simulink model "rasoc_tesis_v4"  (R2021a)
settings: Solver=FixedStepAuto  StartTime=0.0  StopTime=inf  FixedStep=0.01  RelTol=1e-3
values from neighbouring files (symbols this model uses):
  a = 0.445    [param_tesis.m]
  a_max = v_max/dt    (= 0.8)    [param_tesis.m]
  alt_z = 0    [param_tesis.m]
  B = 0.5    [param_tesis.m]
  currentPose = [47 43.5 0]    [param_tesis.m]
  efic_red = 0.95    [param_tesis.m]
  goalPose = [1.5 5 pi/2]    [param_tesis.m]
  gpsBasePose = [1 44]    [param_tesis.m]
  kb = 8.93*(3/(1000*pi))    (= 0.00852752185086)    [param_tesis.m]
  kt = 0.077*sqrt(2)*3    [param_tesis.m]
  L = 0.55    [param_tesis.m]
  m_uva = 0    [param_tesis.m]
  n = 16    [param_tesis.m]
  r = 0.125    [param_tesis.m]
  Ra = Vnom/Ipeak    (= 14.2857142857)    [param_tesis.m]
  Rp = Ra*20    (= 285.714285714)    [param_tesis.m]
  t_lpf = 1/200    (= 0.005)    [param_tesis.m]
  tau_max = 5    [param_tesis.m]
  v_max = 0.8    [param_tesis.m]
  Vnom = 310    [param_tesis.m]
  w_max = 0.5    [param_tesis.m]
  waypoints = [currentPose(1), currentPose(2) ... (first row only)    [AstarHybrid_fn.m]    (also in param_tesis.m = AstarHybrid_fn(currentPose, goalPose))
undefined symbols (not defined in the file or in its folder): angular, DiscIntNeverNeededParam, Earth, linear, startTheta, startX, startY, WGS84
libraries: ros2lib x10, simulink x5, mobileRoboticsTrainingLib x3, robotmobilelib x2, pid_lib x2, robotalgslib x2, aerolibtransform2 x2, dspstat3 x1
(part 2 of 2)

== system rasoc_tesis_v4/Subsystem1/Tensión y Motores/Modulador de Tensión ==
  Va_mL* : Inport
  Va_mR* : Inport  Port=2
  Filtro : StateSpace  A=[-1/t_lpf]  B=[1]  C=[1/t_lpf]  D=[0]  InitialCondition=0
  Filtro PB 1° Orden : StateSpace  A=[-1/t_lpf]  B=[1]  C=[1/t_lpf]  D=[0]  InitialCondition=0
  Saturación : Saturate  UpperLimit=Vnom  LowerLimit=-Vnom
  Saturation : Saturate  UpperLimit=Vnom  LowerLimit=-Vnom
  Va_mL : Outport
  Va_mR : Outport  Port=2
  wires:
  Filtro PB 1° Orden/1 -> Saturación/1
  Filtro/1 -> Saturation/1
  Saturation/1 -> Va_mR/1
  Saturación/1 -> Va_mL/1
  Va_mL*/1 -> Filtro PB 1° Orden/1
  Va_mR*/1 -> Filtro/1

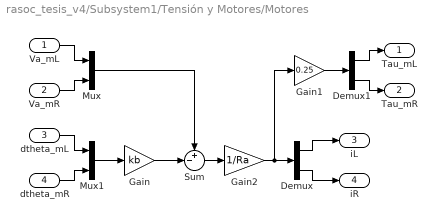
== system rasoc_tesis_v4/Subsystem1/Tensión y Motores/Motores ==
  Va_mL : Inport
  Va_mR : Inport  Port=2
  dtheta_mL : Inport  Port=3
  dtheta_mR : Inport  Port=4
  Demux : Demux  Outputs=2
  Demux1 : Demux  Outputs=2
  Gain : Gain  Gain=kb
  Gain1 : Gain  Gain=0.25
  Gain2 : Gain  Gain=1/Ra
  Mux : Mux  Inputs=2
  Mux1 : Mux  Inputs=2
  Sum : Sum  Inputs=+-|
  Tau_mL : Outport
  Tau_mR : Outport  Port=2
  iL : Outport  Port=3
  iR : Outport  Port=4
  wires:
  Demux/2 -> iR/1
  Va_mL/1 -> Mux/1
  Demux/1 -> iL/1
  dtheta_mR/1 -> Mux1/2
  dtheta_mL/1 -> Mux1/1
  Demux1/2 -> Tau_mR/1
  Demux1/1 -> Tau_mL/1
  Va_mR/1 -> Mux/2
  Mux1/1 -> Gain/1
  Gain1/1 -> Demux1/1
  Gain/1 -> Sum/2
  Mux/1 -> Sum/1
  Sum/1 -> Gain2/1
  Gain2/1 -> Gain1/1, Demux/1

== system rasoc_tesis_v4/Subsystem1/Torque y Corriente/Desacople ==
  Va_mL*' : Inport
  Va_mR*' : Inport  Port=2
  dtheta_mL^ : Inport  Port=3
  dtheta_mR^ : Inport  Port=4
  Demux : Demux  Outputs=2
  Gain1 : Gain  Gain=kb
  Mux : Mux  Inputs=2
  Mux1 : Mux  Inputs=2
  Sum : Sum  Inputs=|++
  Va_mL* : Outport
  Va_mR* : Outport  Port=2
  wires:
  dtheta_mL^/1 -> Mux1/1
  Mux1/1 -> Gain1/1
  Va_mR*'/1 -> Mux/2
  Demux/1 -> Va_mL*/1
  Gain1/1 -> Sum/2
  Mux/1 -> Sum/1
  Sum/1 -> Demux/1
  Va_mL*'/1 -> Mux/1
  Demux/2 -> Va_mR*/1
  dtheta_mR^/1 -> Mux1/2

== system rasoc_tesis_v4/Subsystem1/Torque y Corriente/Modulador de Corriente ==
  "iL* " : Inport
  iR* : Inport  Port=2
  iL^ : Inport  Port=3
  iR^ : Inport  Port=4
  Control Proporcional : Gain  Gain=Rp
  Demux : Demux  Outputs=2
  Mux : Mux  Inputs=2
  Sum : Sum  Inputs=-+|
  Sum1 : Sum  Inputs=|+-
  Va_mL*' : Outport
  Va_mR*' : Outport  Port=2
  wires:
  iL^/1 -> Sum/1
  "iL* "/1 -> Sum/2
  iR*/1 -> Sum1/1
  iR^/1 -> Sum1/2
  Mux/1 -> Control Proporcional/1
  Control Proporcional/1 -> Demux/1
  Sum/1 -> Mux/1
  Sum1/1 -> Mux/2
  Demux/1 -> Va_mL*'/1
  Demux/2 -> Va_mR*'/1

== system rasoc_tesis_v4/Subsystem1/Torque y Corriente/Modulador de Torque ==
  Tau_mL* : Inport
  Tau_mR* : Inport  Port=2
  Demux : Demux  Outputs=2
  Gain : Gain  Gain=1/kt
  Mux : Mux  Inputs=2
  Saturation : Saturate  UpperLimit=tau_max  LowerLimit=-tau_max
  iL* : Outport
  iR* : Outport  Port=2
  wires:
  Tau_mL*/1 -> Mux/1
  Demux/2 -> iR*/1
  Demux/1 -> iL*/1
  Gain/1 -> Demux/1
  Tau_mR*/1 -> Mux/2
  Mux/1 -> Saturation/1
  Saturation/1 -> Gain/1

== system rasoc_tesis_v4/Subsystem4/Local Navigation/Path Following ==
  SteeringDirection : Inport
  AngularVelocity : Inport  Port=2
  Action Port : ActionPort  ActionPortLabel=else
  Compute Angular Velocity : MATLAB Function  TreatAsAtomicUnit=on
  Constant : Constant  Value=0
  MaxAngularVelocity : Constant  Value=w_max
  Subtract : Sum  Inputs=+-
  dV : Outport  VectorParamsAs1DForOutWhenUnconnected=off
  dW : Outport  Port=2  VectorParamsAs1DForOutWhenUnconnected=off
  wires:
  Constant/1 -> dV/1
  MaxAngularVelocity/1 -> Compute Angular Velocity/2(wMax)
  SteeringDirection/1 -> Compute Angular Velocity/1(steeringDir)
  Subtract/1 -> dW/1
  Compute Angular Velocity/1(w) -> Subtract/1
  AngularVelocity/1 -> Subtract/2

== system rasoc_tesis_v4/Subsystem4/Local Navigation/Recovery ==
  LinVel : Inport
  AngVel : Inport  Port=2
  Action Port : ActionPort  ActionPortLabel=if(u1 == 1)
  Constant1 : Constant  Value=0.2
  Gain : Gain  Gain=-1
  Subtract : Sum  Inputs=+-
  dV : Outport  VectorParamsAs1DForOutWhenUnconnected=off
  dW : Outport  Port=2  VectorParamsAs1DForOutWhenUnconnected=off
  wires:
  LinVel/1 -> Gain/1
  Gain/1 -> dV/1
  Constant1/1 -> Subtract/1
  AngVel/1 -> Subtract/2
  Subtract/1 -> dW/1

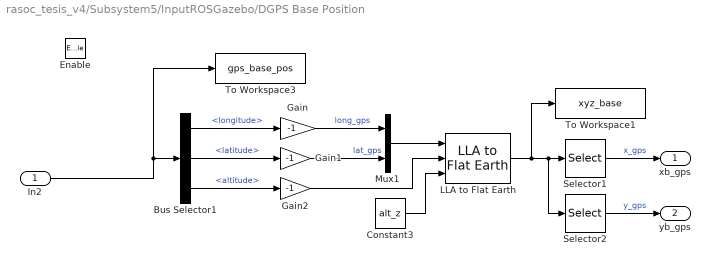
== system rasoc_tesis_v4/Subsystem5/InputROSGazebo/DGPS Base Position ==
  In2 : Inport
  Enable : EnablePort
  Bus Selector1 : BusSelector  OutputSignals=longitude,latitude,altitude
  Constant3 : Constant  Value=alt_z
  Gain : Gain  Gain=-1
  Gain1 : Gain  Gain=-1
  Gain2 : Gain  Gain=-1
  LLA to Flat Earth : aerolibtransform2/LLA to Flat Earth  units=Metric (MKS)  ptype=Earth (WGS84)  F=1/298.257223563  R=6378137  refPosPort=off  LL0=[0 0]  psi=0
      settings: SourceProductBaseCode=AE
  Mux1 : Mux  Inputs=2
  Selector1 : Selector  InputPortWidth=3  IndexOptions=Index vector (dialog)  Indices=[1]  OutputSizes=1
  Selector2 : Selector  InputPortWidth=3  IndexOptions=Index vector (dialog)  Indices=[2]  OutputSizes=1
  To Workspace1 : ToWorkspace  VariableName=xyz_base  SampleTime=-1
  To Workspace3 : ToWorkspace  VariableName=gps_base_pos  SaveFormat=Timeseries  SampleTime=-1
  xb_gps : Outport
  yb_gps : Outport  Port=2
  wires:
  In2/1 -> Bus Selector1/1, To Workspace3/1
  Bus Selector1/2 -> Gain1/1  "<latitude>"
  Bus Selector1/1 -> Gain/1  "<longitude>"
  Gain2/1 -> LLA to Flat Earth/2
  Mux1/1 -> LLA to Flat Earth/1
  LLA to Flat Earth/1 -> Selector2/1, Selector1/1, To Workspace1/1
  Gain/1 -> Mux1/1  "long_gps"
  Gain1/1 -> Mux1/2  "lat_gps"
  Constant3/1 -> LLA to Flat Earth/3
  Bus Selector1/3 -> Gain2/1  "<altitude>"
  Selector1/1 -> xb_gps/1  "x_gps"
  Selector2/1 -> yb_gps/1  "y_gps"

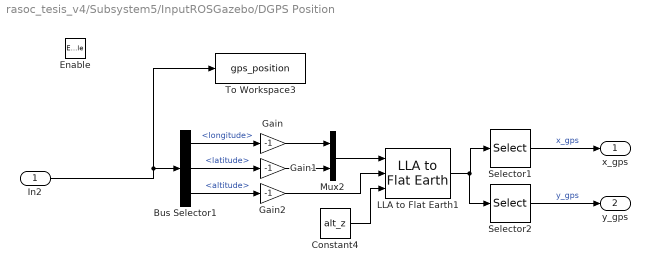
== system rasoc_tesis_v4/Subsystem5/InputROSGazebo/DGPS Position ==
  In2 : Inport
  Enable : EnablePort
  Bus Selector1 : BusSelector  OutputSignals=longitude,latitude,altitude
  Constant4 : Constant  Value=alt_z
  Gain : Gain  Gain=-1
  Gain1 : Gain  Gain=-1
  Gain2 : Gain  Gain=-1
  LLA to Flat Earth1 : aerolibtransform2/LLA to Flat Earth  units=Metric (MKS)  ptype=Earth (WGS84)  F=1/298.257223563  R=6378137  refPosPort=off  LL0=[0 0]  psi=0
      settings: SourceProductBaseCode=AE
  Mux2 : Mux  Inputs=2
  Selector1 : Selector  InputPortWidth=3  IndexOptions=Index vector (dialog)  Indices=[1]  OutputSizes=1
  Selector2 : Selector  InputPortWidth=3  IndexOptions=Index vector (dialog)  Indices=[2]  OutputSizes=1
  To Workspace3 : ToWorkspace  VariableName=gps_position  SaveFormat=Timeseries  SampleTime=-1
  x_gps : Outport
  y_gps : Outport  Port=2
  wires:
  Bus Selector1/1 -> Gain/1  "<longitude>"
  Bus Selector1/2 -> Gain1/1  "<latitude>"
  In2/1 -> To Workspace3/1, Bus Selector1/1
  Bus Selector1/3 -> Gain2/1  "<altitude>"
  Constant4/1 -> LLA to Flat Earth1/3
  Mux2/1 -> LLA to Flat Earth1/1
  Gain2/1 -> LLA to Flat Earth1/2
  Gain1/1 -> Mux2/2
  Gain/1 -> Mux2/1
  LLA to Flat Earth1/1 -> Selector2/1, Selector1/1
  Selector1/1 -> x_gps/1  "x_gps"
  Selector2/1 -> y_gps/1  "y_gps"

== system rasoc_tesis_v4/Subsystem5/InputROSGazebo/DGPS Vel ==
  In1 : Inport
  Enable : EnablePort
  Bus Selector3 : BusSelector  OutputSignals=vector.x,vector.y
  Gain : Gain  Gain=-1
  Gain1 : Gain  Gain=-1
  To Workspace6 : ToWorkspace  VariableName=gps_velocity  SaveFormat=Timeseries  SampleTime=-1
  dx_gps : Outport
  dy_gps : Outport  Port=2
  wires:
  Bus Selector3/1 -> Gain/1  "<x>"
  In1/1 -> To Workspace6/1, Bus Selector3/1
  Bus Selector3/2 -> Gain1/1  "<y>"
  Gain/1 -> dx_gps/1
  Gain1/1 -> dy_gps/1

== system rasoc_tesis_v4/Subsystem5/InputROSGazebo/GPS2ROS ==
  x_gps : Inport
  y_gps : Inport  Port=2
  v_gps : Inport  Port=3
  w_gps : Inport  Port=4
  Action Port : ActionPort  ActionPortLabel=if(u1 == 1)
  x_ros : Outport  VectorParamsAs1DForOutWhenUnconnected=off
  y_ros : Outport  Port=2  VectorParamsAs1DForOutWhenUnconnected=off
  v_ros : Outport  Port=3  VectorParamsAs1DForOutWhenUnconnected=off
  w_ros : Outport  Port=4  VectorParamsAs1DForOutWhenUnconnected=off
  wires:
  x_gps/1 -> x_ros/1
  y_gps/1 -> y_ros/1
  w_gps/1 -> w_ros/1
  v_gps/1 -> v_ros/1

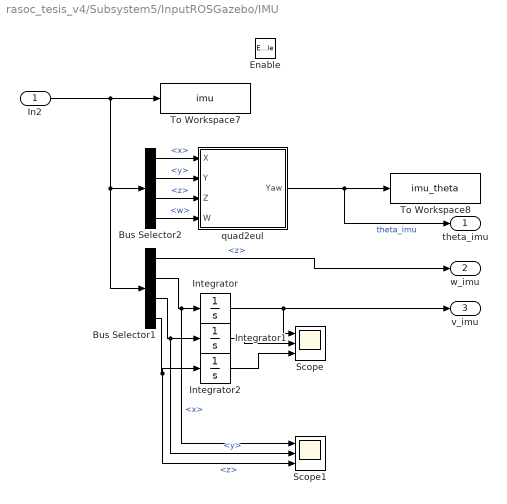
== system rasoc_tesis_v4/Subsystem5/InputROSGazebo/IMU ==
  In2 : Inport
  Enable : EnablePort
  Bus Selector1 : BusSelector  OutputSignals=angular_velocity.z,linear_acceleration.x,linear_acceleration.y,linear_acceleration.z
  Bus Selector2 : BusSelector  OutputSignals=orientation.x,orientation.y,orientation.z,orientation.w
  Integrator : Integrator
  Integrator1 : Integrator
  Integrator2 : Integrator
  Scope : Scope  NumInputPorts=3
  Scope1 : Scope  NumInputPorts=3
  To Workspace7 : ToWorkspace  VariableName=imu  SaveFormat=Timeseries  SampleTime=-1
  To Workspace8 : ToWorkspace  VariableName=imu_theta  SaveFormat=Timeseries  SampleTime=-1
  quad2eul : MATLAB Function  TreatAsAtomicUnit=on
  theta_imu : Outport
  w_imu : Outport  Port=2
  v_imu : Outport  Port=3
  wires:
  Bus Selector2/3 -> quad2eul/3(Z)  "<z>"
  quad2eul/1(Yaw) -> theta_imu/1, To Workspace8/1  "theta_imu"
  In2/1 -> Bus Selector1/1, Bus Selector2/1, To Workspace7/1
  Bus Selector2/1 -> quad2eul/1(X)  "<x>"
  Bus Selector2/4 -> quad2eul/4(W)  "<w>"
  Bus Selector2/2 -> quad2eul/2(Y)  "<y>"
  Bus Selector1/1 -> w_imu/1  "<z>"
  Bus Selector1/2 -> Scope1/1, Integrator/1  "<x>"
  Integrator/1 -> Scope/1, v_imu/1
  Bus Selector1/3 -> Scope1/2, Integrator1/1  "<y>"
  Bus Selector1/4 -> Scope1/3, Integrator2/1  "<z>"
  Integrator1/1 -> Scope/2
  Integrator2/1 -> Scope/3

== system rasoc_tesis_v4/Subsystem5/InputROSGazebo/IMU2ROS ==
  theta_imu : Inport
  Action Port : ActionPort  ActionPortLabel=if(u1 == 1)
  theta_ros : Outport  VectorParamsAs1DForOutWhenUnconnected=off
  wires:
  theta_imu/1 -> theta_ros/1

== system rasoc_tesis_v4/Subsystem5/InputROSGazebo/LIDAR ==
  In1 : Inport
  MATLAB Function : MATLAB Function  TreatAsAtomicUnit=on
  To Workspace1 : ToWorkspace  VariableName=Lidar  SaveFormat=Timeseries  SampleTime=-1
  Ranges : Outport
  Angles : Outport  Port=2
  wires:
  In1/1 -> To Workspace1/1, MATLAB Function/1(LaserScanMsg)
  MATLAB Function/2(Angles) -> Angles/1
  MATLAB Function/1(Ranges) -> Ranges/1

== system rasoc_tesis_v4/Subsystem5/InputROSGazebo/ODOM2ROS ==
  x_odom : Inport
  y_odom : Inport  Port=2
  v_odom : Inport  Port=3
  w_odom : Inport  Port=4
  Action Port : ActionPort  ActionPortLabel=else
  x_ros : Outport  VectorParamsAs1DForOutWhenUnconnected=off
  y_ros : Outport  Port=2  VectorParamsAs1DForOutWhenUnconnected=off
  v_ros : Outport  Port=3  VectorParamsAs1DForOutWhenUnconnected=off
  w_ros : Outport  Port=4  VectorParamsAs1DForOutWhenUnconnected=off
  wires:
  x_odom/1 -> x_ros/1
  y_odom/1 -> y_ros/1
  v_odom/1 -> v_ros/1
  w_odom/1 -> w_ros/1

== system rasoc_tesis_v4/Subsystem5/InputROSGazebo/ODOM2ROS_theta ==
  theta_odom : Inport
  Action Port : ActionPort  ActionPortLabel=else
  theta_ros : Outport  VectorParamsAs1DForOutWhenUnconnected=off
  wires:
  theta_odom/1 -> theta_ros/1

== system rasoc_tesis_v4/Subsystem5/InputROSGazebo/Odometry ==
  In1 : Inport
  Bus Selector : BusSelector  OutputSignals=pose.pose.position.x,pose.pose.position.y,pose.pose.orientation.x,pose.pose.orientation.y,pose.pose.orientation.z,pose.pose.orientation.w
  Bus Selector1 : BusSelector  OutputSignals=twist.twist.linear.x,twist.twist.angular.z
  XY ODOM : simulink/Sinks/XY Graph  Commented=on  xmin=0  xmax=50  ymin=-5  ymax=50  st=-1
  quad2eul : MATLAB Function  TreatAsAtomicUnit=on
  x_odom : Outport
  y_odom : Outport  Port=2
  theta_odom : Outport  Port=3
  v_odom : Outport  Port=4
  w_odom : Outport  Port=5
  wires:
  Bus Selector/5 -> quad2eul/3(Z)  "<z>"
  Bus Selector/1 -> x_odom/1, XY ODOM/1  "<x>"
  quad2eul/1(Yaw) -> theta_odom/1
  Bus Selector/3 -> quad2eul/1(X)  "<x>"
  Bus Selector1/1 -> v_odom/1  "<x>"
  Bus Selector/2 -> y_odom/1, XY ODOM/2  "<y>"
  In1/1 -> Bus Selector/1, Bus Selector1/1
  Bus Selector1/2 -> w_odom/1  "<z>"
  Bus Selector/6 -> quad2eul/4(W)  "<w>"
  Bus Selector/4 -> quad2eul/2(Y)  "<y>"

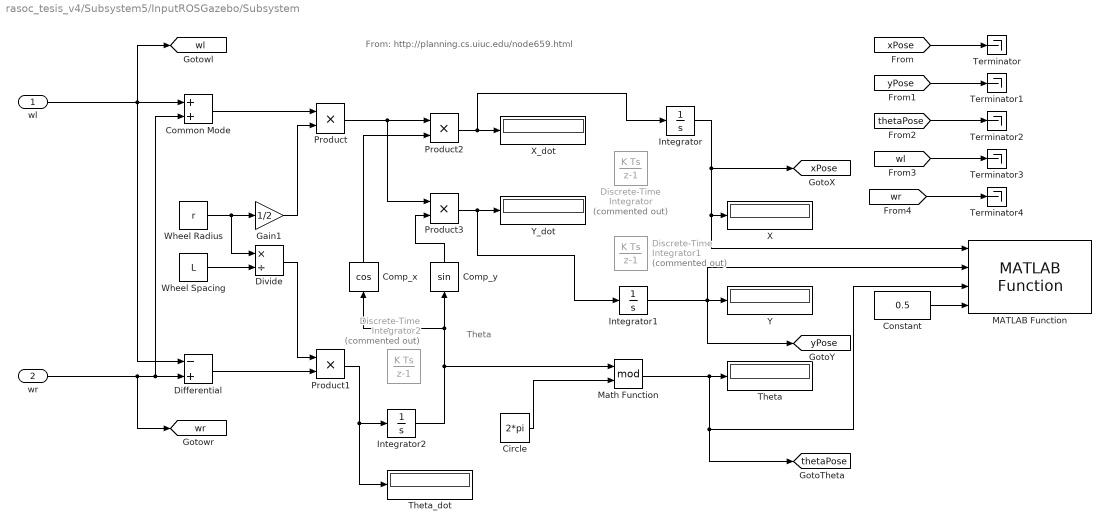
== system rasoc_tesis_v4/Subsystem5/InputROSGazebo/Subsystem ==
  note: Theta
  note: From: http://planning.cs.uiuc.edu/node659.html
  wl : Inport
  wr : Inport  Port=2
  Circle : Constant  Value=2*pi
  Common Mode : Sum
  Comp_x : Trigonometry  Operator=cos
  Comp_y : Trigonometry
  Constant : Constant  Value=0.5
  Differential : Sum  Inputs=-+
  Discrete-Time Integrator : DiscreteIntegrator  Commented=on  InitialCondition=startX  SampleTime=-1  ICPrevOutput=DiscIntNeverNeededParam  ICPrevScaledInput=DiscIntNeverNeededParam
  Discrete-Time Integrator1 : DiscreteIntegrator  Commented=on  InitialCondition=startY  SampleTime=-1  ICPrevOutput=DiscIntNeverNeededParam  ICPrevScaledInput=DiscIntNeverNeededParam
  Discrete-Time Integrator2 : DiscreteIntegrator  Commented=on  InitialCondition=startTheta*(pi/180)  SampleTime=-1  ICPrevOutput=DiscIntNeverNeededParam  ICPrevScaledInput=DiscIntNeverNeededParam
  Divide : Product  Inputs=*/
  Gain1 : Gain  Gain=1/2
  Integrator : Integrator  InitialCondition=currentPose(1)
  Integrator1 : Integrator  InitialCondition=currentPose(2)
  Integrator2 : Integrator  InitialCondition=currentPose(3)
  MATLAB Function : mobileRoboticsTrainingLib/Robot Simulator/MATLAB Function  SystemSampleTime=-1  VariantActivationTime=update diagram  Latency=0  AutoFrameSizeCalculation=off
      settings: SourceProductName=Mobile Robotics Training Library
  Math Function : Math  Operator=mod  SignedPower=on  SaturateOnIntegerOverflow=on
  Product{,1..3} (4 alike) : Product  RndMeth=Zero
  Terminator{,1..4} (5 alike) : Terminator
  Theta : Display
  Theta_dot : Display
  Wheel Radius : Constant  Value=r
  Wheel Spacing : Constant  Value=L
  X : Display
  X_dot : Display
  Y : Display
  Y_dot : Display
  tag scope: thetaPose=global, wl=global, wr=global, xPose=global, yPose=global
  wires:
  Common Mode/1 -> Product/1
  Math Function/1 -> [thetaPose], MATLAB Function/3, Theta/1
  wl/1 -> [wl], Common Mode/1, Differential/1
  Integrator2/1 -> Math Function/1, Comp_x/1, Comp_y/1
  Divide/1 -> Product1/1
  Product3/1 -> Integrator1/1, Y_dot/1
  Wheel Radius/1 -> Divide/1, Gain1/1
  Integrator/1 -> [xPose], MATLAB Function/1, X/1
  Wheel Spacing/1 -> Divide/2
  [wr] -> Terminator4/1
  Comp_y/1 -> Product3/2
  Differential/1 -> Product1/2
  wr/1 -> [wr], Common Mode/2, Differential/2
  Product/1 -> Product3/1, Product2/1
  Product2/1 -> Integrator/1, X_dot/1
  Gain1/1 -> Product/2
  Comp_x/1 -> Product2/2
  [thetaPose] -> Terminator2/1
  Integrator1/1 -> MATLAB Function/2, Y/1, [yPose]
  Constant/1 -> MATLAB Function/4
  Circle/1 -> Math Function/2
  [wl] -> Terminator3/1
  Product1/1 -> Integrator2/1, Theta_dot/1
  [yPose] -> Terminator1/1
  [xPose] -> Terminator/1

== system rasoc_tesis_v4/Subsystem5/InputROSGazebo/vw2wLwR ==
  v_ros : Inport
  w_ros : Inport  Port=2
  Gain10 : Gain  Gain=1/r
  Gain8 : Gain  Gain=L/2
  Gain9 : Gain  Gain=1/r
  Sum7 : Sum  Inputs=|+-
  Sum8 : Sum  Inputs=++|
  wL_ros : Outport
  wR_ros : Outport  Port=2
  wires:
  Sum8/1 -> Gain10/1
  w_ros/1 -> Gain8/1
  Gain8/1 -> Sum7/2, Sum8/2
  Gain10/1 -> wR_ros/1
  Sum7/1 -> Gain9/1
  v_ros/1 -> Sum7/1, Sum8/1
  Gain9/1 -> wL_ros/1

== matlab function rasoc_tesis_v4/Subsystem1/Dinamica Directa/MATLAB Function ==
  data: tauRu_L input; ddthetaL output; tauRu_R input; ddthetaR output; M_ag input; tauFr input; alfa input
function [ddthetaL, ddthetaR] = din_dir (tauRu_L, tauRu_R, M_ag, tauFr,alfa)
%% Geometría del Robot
a = 0.445;      %%% Distancia del Eje Motriz al Centro de Masa
L = 0.55;       %%% Separación entre ruedas
r = 0.125;      %%% Radio de Rueda Motriz
length = 1.25;
width = 0.75;
height = 0.79;

%% Dinámica
M = 65 + M_ag;
mg = 1.5;
mc = 1;
I = M*(length^2 + width^2)/12;
alfa_rad = alfa*pi/180;
g = 9.81;

tau = [tauRu_R; tauRu_L];   %%% Vector de Torques
tau = tau - tauFr;          %%% Resto el Torque de Fricción

%% Versión CyS
c1 = (M*r^2)/2;     c2 = 1/4;   c3 = a/L;   c4 = I/(M*L^2);     c5 = (r^2)*(3*mc+2*mg);
D = 2*c1*[c2+c3+c4+(c5/c1)        c2-c4;
            c2-c4           c2+c3+c4+(c5/c1)];

%% Cálculo de Aceleraciones
tau_p = (r/2)*M*g*sin(alfa_rad)*[1;1];  %Torques de pendiente de 30 grados
tau = tau - tau_p;
ddtheta = D\tau;            %%% Inversa de D * Tau
ddthetaL = ddtheta(2); 
ddthetaR = ddtheta(1);

== matlab function rasoc_tesis_v4/Subsystem5/InputROSGazebo/LIDAR/MATLAB Function ==
  data: LaserScanMsg input; Ranges output; Angles output
function [Ranges, Angles] = ExtractRangeData(LaserScanMsg)
%#codegen

% Extract Range information
Ranges = double(LaserScanMsg.ranges);

% Construct Angles vector using AngleMin and AngleIncrement from sensor
% reading.
angMin = double(LaserScanMsg.angle_min);
angIncrement = double(LaserScanMsg.angle_increment);

numReadings = numel(Ranges);
Angles = angMin + (0:numReadings-1)' * angIncrement;

% Wrap the angles to the (-pi,pi] interval.
% Angles = robotics.internal.wrapToPi(double(rawAngles));

== matlab function rasoc_tesis_v4/Subsystem1/Dinamica Inversa/MATLAB Function ==
  data: ddthetaL input; tauTot_L output; ddthetaR input; tauTot_R output; M_ag input
function [tauTot_L, tauTot_R] = din_inv(ddthetaL, ddthetaR, M_ag)
%% Geometría del Robot
a = 0.445;      %%% Distancia del Eje Motriz al Centro de Masa
L = 0.55;       %%% Separación entre ruedas
r = 0.125;      %%% Radio de Rueda Motriz
length = 1.25;
width = 0.75;
height = 0.79;

%% Dinámica
M = 65 + M_ag;
mg = 1.5;
mc = 1;
I = M*(length^2 + width^2)/12;

ddtheta = [ddthetaR; ddthetaL]; %Vector de aceleraciones

%% Versión CyS
c1 = (M*r^2)/2;     c2 = 1/4;   c3 = a/L;   c4 = I/(M*L^2);     c5 = (r^2)*(2*mc+mg);
D = 2*c1*[c2+c3+c4+(c5/c1)        c2-c4;
            c2-c4           c2+c3+c4+(c5/c1)];

%% Cálculo de Torques
tau = D*ddtheta;     

tauTot = tau;
tauTot_L = tauTot(2); 
tauTot_R = tauTot(1);

== matlab function rasoc_tesis_v4/Subsystem5/InputROSGazebo/Odometry/quad2eul ==
  data: X input; Yaw output; Y input; Z input; W input
function Yaw = quat2eulBlk(X, Y, Z, W)
%#codegen

eularAngles = quat2eul([W, X, Y, Z]);
Yaw = eularAngles(1); %eulerAngles=[z,y,x]

== matlab function rasoc_tesis_v4/Subsystem4/Local Navigation/Path Following/Compute Angular Velocity ==
  data: steeringDir input; w output; wMax input
function w = exampleHelperComputeAngularVelocity(steeringDir, wMax)
%EXAMPLEHELPERCOMPUTEANGULARVELOCITY Compute angular velocity
%   W = exampleHelperComputeAngularVelocity(STEERINGDIR)
%   returns the angular velocity W for a differential drive robot in radians
%   per second for a given steering direction STEERINGDIR in the robot's
%   coordinate frame in radians.
%
%   W = exampleHelperComputeAngularVelocity(STEERINGDIR, WMAX)
%   returns the angular velocity W for a differential drive robot in radians
%   per second for a given steering direction STEERINGDIR in the robot's
%   coordinate frame in radians and maximum angular velocity WMAX in
%   radians per second. The output angular velocity is saturated based on
%   the WMAX.
%
%   Example:
%       
%       w = exampleHelperComputeAngularVelocity(0.2, 1);

% Copyright 2015 The MathWorks, Inc.

%#codegen
%#ok<*EMCA>

% Allow variable input arguments
if nargin == 1   
    wMax = inf;
end

validateattributes(steeringDir, {'double'},{'real'},...
    'exampleHelperComputeAngularVelocity', 'STEERINGDIR', 1);
validateattributes(wMax, {'double'},{'real', 'positive'},...
    'exampleHelperComputeAngularVelocity', 'WMAX', 2);

% Computing in robot's coordinate frame
curPose = [0 0 0];

% The following computation is similar to robotics.PurePursuit
lookaheadPoint = [cos(steeringDir), sin(steeringDir)];
slope = atan2((lookaheadPoint(2) - curPose(2)), ...
    (lookaheadPoint(1) - curPose(1)));
alpha = angdiff(curPose(3), slope);

% Angular velocity command for a differential drive robot is
% equal to the desired curvature to be followed by the robot.

w = (2*sin(alpha));

% Pick a constant rotation when robot is facing in the opposite
% direction of the path
if abs(abs(alpha) - pi) < 1e-12
    w = sign(w)*1;
end

if abs(w) > wMax
    w = sign(w)*wMax;
end

end

== matlab function rasoc_tesis_v4/Subsystem5/InputROSGazebo/IMU/quad2eul ==
  data: X input; Yaw output; Y input; Z input; W input
function Yaw = quat2euler(X, Y, Z, W)
%#codegen

eularAngles = quat2eul([W, X, Y, Z]);
Yaw = eularAngles(1); %eulerAngles=[z,y,x]

== matlab function rasoc_tesis_v4/Subsystem5/InputROSGazebo/MATLAB Function ==
  data: dx input; dy input; theta input; v output; dtheta input; w output; a input
function [v, w] = vw2xy(dx, dy, theta, dtheta, a)
P = [  dx; 
       dy;
     dtheta];
J = [cos(theta), -a*sin(theta);
     sin(theta),  a*cos(theta);
         0     ,       1      ];
     
V = J\P;
v = V(1);
w = V(2);
